simulink model "lab4_sim"  (R2017a)
settings: Solver=FixedStepAuto  StartTime=0.0  StopTime=2  FixedStep=T  RelTol=1e-3
values from neighbouring files (symbols this model uses):
  A = [0 1 0 0; Amat 0 0 -((Amat*Cmat)/(n*g)); 0 0 0 1; 0 0 0 -Cmat]    [lab4_Prelim.m]    (also in lab4_Robust.m)
  A_obs = (phi - L*C - gamma*K)    [lab4_Prelim.m]    (also in lab4_Robust.m)
  B = [0; ((Amat*D)/(n*g)); 0; D]    [lab4_Prelim.m]    (also in lab4_Robust.m)
  B_obs = L    [lab4_Prelim.m]    (also in lab4_Robust.m)
  C = [1 0 0 0; 0 0 1 0]    [lab4_Prelim.m]    (also in lab4_Robust.m)
  C_obs = -K    [lab4_Prelim.m]    (also in lab4_Robust.m)
  D_obs = [0 0]    [lab4_Prelim.m]    (also in lab4_Robust.m)
  q = 10^(0.21/20)    (= 1.02447178031)    [lab4_Prelim.m]    (also in lab4_Robust.m)
  T = 0.01    [lab4_Prelim.m]    (also in lab4_Robust.m)
  x0 = [0.17; 0; 0; 0]    [lab4_Prelim.m]    (also in lab4_Robust.m)
  x0_obs = C\(C*x0)    [lab4_Prelim.m]    (also in lab4_Robust.m)
settings Model: Creator=njohnson  LastModifiedBy=njohnson

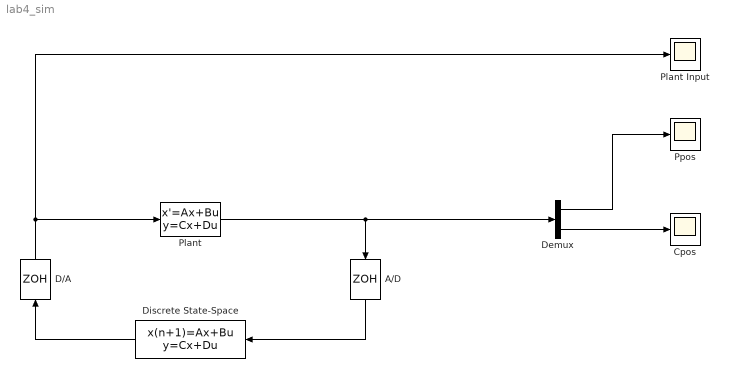
== system lab4_sim ==
  A/D : ZeroOrderHold  SampleTime=T
  "Cpos " : Scope
  D/A : ZeroOrderHold  SampleTime=T
  Demux : Demux  Outputs=2
  Discrete State-Space : DiscreteStateSpace  A=A_obs  B=B_obs  C=C_obs  D=D_obs  X0=x0_obs  SampleTime=T
  Plant : StateSpace  A=A  B=q*B  C=C  D=[0; 0]  X0=x0
  "Plant Input " : Scope
  "Ppos " : Scope
  wires:
  D/A/1 -> Plant/1, "Plant Input "/1
  Plant/1 -> Demux/1, A/D/1
  A/D/1 -> Discrete State-Space/1
  Demux/1 -> "Ppos "/1
  Demux/2 -> "Cpos "/1
  Discrete State-Space/1 -> D/A/1
